simulink model "HRBModel"  (R2021b)
settings: Solver=VariableStepAuto  StartTime=0.0  StopTime=T_sim  RelTol=1e-3
values from neighbouring files (symbols this model uses):
  A = 7.20598    [HRBData.sldd]    (also in HRBModelParam.m = 7.20598)
  A_Tank = 0.25    [HRBData.sldd]    (also in HRBModelParam.m = 0.25)
  act_time = 10.0    [HRBData.sldd]    (also in HRBModelParam.m = 10)
  alpha = 0.0    [HRBData.sldd]    (also in HRBModelParam.m = deg2rad(0))
  Cd = 0.8    [HRBData.sldd]    (also in HRBModelParam.m = 0.8)
  Cr = 0.018    [HRBData.sldd]    (also in HRBModelParam.m = 0.018)
  DV = 80.0    [HRBData.sldd]    (also in HRBModelParam.m = 80)
  g = 9.81    [HRBData.sldd]    (also in HRBModelParam.m = 9.81)
  gamma = 1.4    [HRBData.sldd]    (also in HRBModelParam.m = 1.4)
  ilk_hiz = 15.0    [HRBData.sldd]    (also in HRBModelParam.m = 0)
  m = 18000.0    [HRBData.sldd]    (also in HRBModelParam.m = 18000)
  mech_eff = 0.9    [HRBData.sldd]    (also in HRBModelParam.m = 0.9)
  mu_AT = 0.8    [HRBData.sldd]    (also in HRBModelParam.m = 0.8)
  mu_HA = 0.8    [HRBData.sldd]    (also in HRBModelParam.m = 0.8)
  P0 = 50.0    [HRBData.sldd]    (also in HRBModelParam.m = 50)
  P1 = 60.0    [HRBData.sldd]    (also in HRBModelParam.m = 395)
  Patm = 1.0    [HRBData.sldd]    (also in HRBModelParam.m = 1)
  Pmax = 400.0    [HRBData.sldd]    (also in HRBModelParam.m = 400)
  r = 0.5715    [HRBData.sldd]    (also in HRBModelParam.m = 0.5715)
  R_AT = 4.11    [HRBData.sldd]    (also in HRBModelParam.m = 4.11)
  R_HA = 7.0    [HRBData.sldd]    (also in HRBModelParam.m = 7)
  R_PM_Aku = 0.07    [HRBData.sldd]    (also in HRBModelParam.m = 0.07)
  rho = 1.225    [HRBData.sldd]    (also in HRBModelParam.m = 1.225)
  rho_oil = 700.0    [HRBData.sldd]    (also in HRBModelParam.m = 700)
  V0 = 0.06    [HRBData.sldd]    (also in HRBModelParam.m = 0.06)
  V_oil = 0.1    [HRBData.sldd]    (also in HRBModelParam.m = 0.1)
  vol_eff = 0.9    [HRBData.sldd]    (also in HRBModelParam.m = 0.9)
libraries: simulink_extras x1
settings Model: DataDictionary=HRBData.sldd  Creator=erkin  LastModifiedBy=erkin

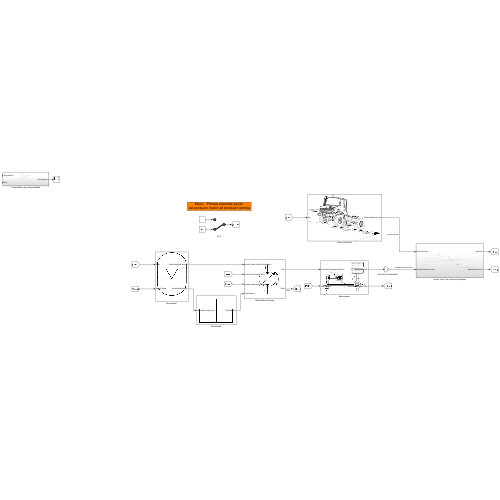
[thumbnail: Simulink's stored preview of the top-level diagram]
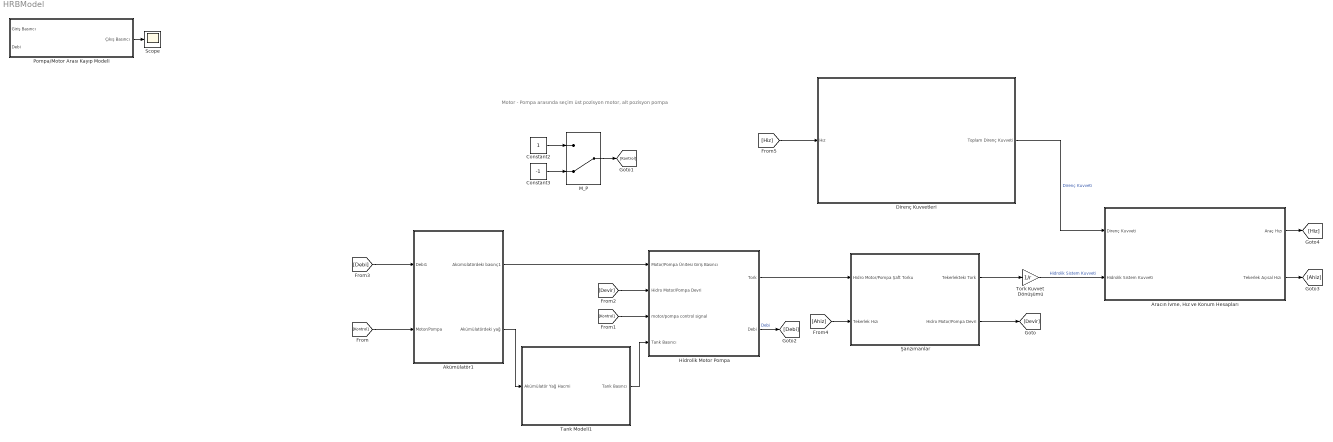
== system HRBModel ==
  note: Motor - Pompa arasında seçim
      | üst pozisyon motor, alt pozisyon pompa
  " Aracın İvme, Hız ve Konum Hesapları" : Subsystem
  Akümülatör1 : Subsystem
      mask Display: image('$imagefile'); % Use "Edit Image" on toolstrip to change.
  Constant2 : Constant
  Constant3 : Constant  Value=-1
  Direnç Kuvvetleri : Subsystem
      mask Display: image('$imagefile'); % Use "Edit Image" on toolstrip to change.
  Hidrolik Motor Pompa : Subsystem
      mask Display: image('$imagefile'); % Use "Edit Image" on toolstrip to change.
  M_P : ManualSwitch  CurrentSetting=0
  Pompa/Motor Arası Kayıp Modeli : Subsystem
  Scope : Scope
  Tank Modeli1 : Subsystem
      mask Display: image('$imagefile'); % Use "Edit Image" on toolstrip to change.
  Tork Kuvvet Dönüşümü : Gain  Gain=1/r
  Şanzımanlar : Subsystem
      mask Display: image('$imagefile'); % Use "Edit Image" on toolstrip to change.
  wires:
  Hidrolik Motor Pompa/1(Tork) -> Şanzımanlar/1(Hidro Motor/Pompa Şaft Torku)
  Şanzımanlar/1(Tekerlekteki Tork) -> Tork Kuvvet Dönüşümü/1
  Tork Kuvvet Dönüşümü/1 -> " Aracın İvme, Hız ve Konum Hesapları"/2(Hidrolik Sistem Kuvveti)  "Hidrolik Sistem Kuvveti"
  Direnç Kuvvetleri/1(Toplam Direnç Kuvveti) -> " Aracın İvme, Hız ve Konum Hesapları"/1(Direnç Kuvveti)  "Direnç Kuvveti"
  [Kontrol] -> Akümülatör1/2(Motor/Pompa)
  Constant2/1 -> M_P/1
  Constant3/1 -> M_P/2
  M_P/1 -> [Kontrol]
  [Kontrol] -> Hidrolik Motor Pompa/3(motor/pompa control signal)
  Tank Modeli1/1(Tank Basıncı) -> Hidrolik Motor Pompa/4(Tank Basıncı)
  Akümülatör1/2("Akümülatördeki yağ ") -> Tank Modeli1/1(Akümülatör Yağ Hacmi)
  Akümülatör1/1(Akümülatördeki basınç1) -> Hidrolik Motor Pompa/1(Motor/Pompa Ünitesi Giriş Basıncı)
  Pompa/Motor Arası Kayıp Modeli/1(Çıkış Basıncı) -> Scope/1
  [Devir] -> Hidrolik Motor Pompa/2(Hidro Motor/Pompa Devri)
  Şanzımanlar/2(Hidro Motor/Pompa Devri) -> [Devir]
  [Debi] -> Akümülatör1/1(Debi1)
  Hidrolik Motor Pompa/2(Debi) -> [Debi]  "Debi"
  " Aracın İvme, Hız ve Konum Hesapları"/2(Tekerlek Açısal Hızı) -> [Ahiz]
  [Ahiz] -> Şanzımanlar/2(Tekerlek Hızı)
  [Hiz] -> Direnç Kuvvetleri/1(Hız)
  " Aracın İvme, Hız ve Konum Hesapları"/1(Araç Hızı) -> [Hiz]

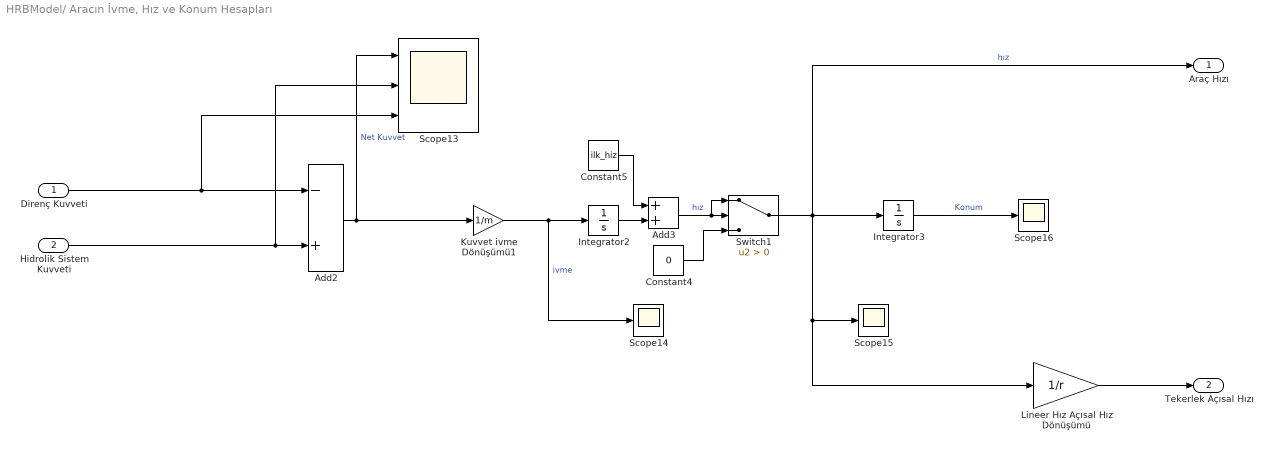
== system HRBModel/ Aracın İvme, Hız ve Konum Hesapları ==
  Direnç Kuvveti : Inport
  Hidrolik Sistem Kuvveti : Inport  Port=2
  Add2 : Sum  Inputs=-+
  Add3 : Sum
  Constant4 : Constant  Value=0
  Constant5 : Constant  Value=ilk_hiz
  Integrator2 : Integrator
  Integrator3 : Integrator
  Kuvvet ivme Dönüşümü1 : Gain  Gain=1/m
  Lineer Hız Açısal Hız Dönüşümü : Gain  Gain=1/r
  Scope13 : Scope  NumInputPorts=3
  Scope14 : Scope
  Scope15 : Scope
  Scope16 : Scope
  Switch1 : Switch  Criteria=u2 > Threshold
  Araç Hızı : Outport
  Tekerlek Açısal Hızı : Outport  Port=2
  wires:
  Kuvvet ivme Dönüşümü1/1 -> Integrator2/1, Scope14/1  "ivme"
  Constant4/1 -> Switch1/3
  Add2/1 -> Kuvvet ivme Dönüşümü1/1, Scope13/1  "Net Kuvvet"
  Integrator2/1 -> Add3/2
  Constant5/1 -> Add3/1
  Switch1/1 -> Araç Hızı/1, Integrator3/1, Lineer Hız Açısal Hız Dönüşümü/1, Scope15/1  "hız"
  Integrator3/1 -> Scope16/1  "Konum"
  Add3/1 -> Switch1/1, Switch1/2  "hız"
  Direnç Kuvveti/1 -> Scope13/3, Add2/1
  Hidrolik Sistem Kuvveti/1 -> Scope13/2, Add2/2
  Lineer Hız Açısal Hız Dönüşümü/1 -> Tekerlek Açısal Hızı/1

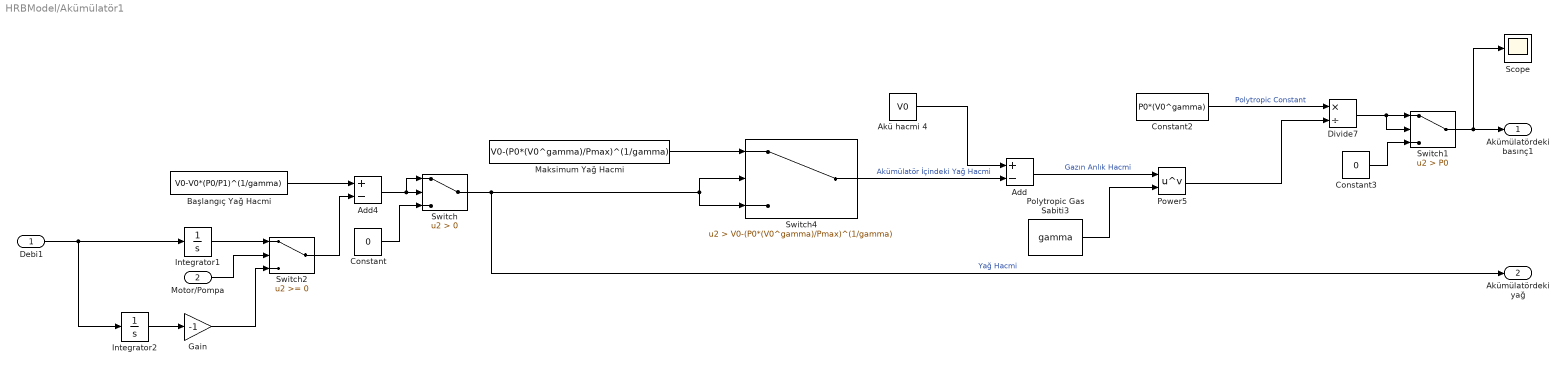
== system HRBModel/Akümülatör1 ==
  Debi1 : Inport
  Motor/Pompa : Inport  Port=2
  Add : Sum  Inputs=+-
  Add4 : Sum  Inputs=+-
  Akü hacmi 4 : Constant  Value=V0
  Başlangıç Yağ Hacmi : Constant  Value=V0-V0*(P0/P1)^(1/gamma)
  Constant : Constant  Value=0
  Constant2 : Constant  Value=P0*(V0^gamma)
  Constant3 : Constant  Value=0
  Divide7 : Product  Inputs=*/
  Gain : Gain  Gain=-1
  Integrator1 : Integrator
  Integrator2 : Integrator
  Maksimum Yağ Hacmi : Constant  Value=V0-(P0*(V0^gamma)/Pmax)^(1/gamma)
  Polytropic Gas Sabiti3 : Constant  Value=gamma
  Power5 : Math  Operator=pow  SaturateOnIntegerOverflow=on
  Scope : Scope
  Switch : Switch  Criteria=u2 > Threshold
  Switch1 : Switch  Criteria=u2 > Threshold  Threshold=P0
  Switch2 : Switch
  Switch4 : Switch  Criteria=u2 > Threshold  Threshold=V0-(P0*(V0^gamma)/Pmax)^(1/gamma)
  Akümülatördeki basınç1 : Outport
  "Akümülatördeki yağ " : Outport  Port=2
  wires:
  Divide7/1 -> Switch1/2, Switch1/1
  Başlangıç Yağ Hacmi/1 -> Add4/1
  Constant2/1 -> Divide7/1  "Polytropic Constant"
  Switch/1 -> "Akümülatördeki yağ "/1, Switch4/2, Switch4/3  "Yağ Hacmi"
  Debi1/1 -> Integrator2/1, Integrator1/1
  Akü hacmi 4/1 -> Add/1
  Add/1 -> Power5/1  "Gazın Anlık Hacmi"
  Polytropic Gas Sabiti3/1 -> Power5/2
  Power5/1 -> Divide7/2
  Add4/1 -> Switch/1, Switch/2
  Constant/1 -> Switch/3
  Constant3/1 -> Switch1/3
  Integrator1/1 -> Switch2/1
  Switch2/1 -> Add4/2
  Integrator2/1 -> Gain/1
  Gain/1 -> Switch2/3
  Switch1/1 -> Scope/1, Akümülatördeki basınç1/1
  Motor/Pompa/1 -> Switch2/2
  Maksimum Yağ Hacmi/1 -> Switch4/1
  Switch4/1 -> Add/2  "Akümülatör İçindeki Yağ Hacmi"

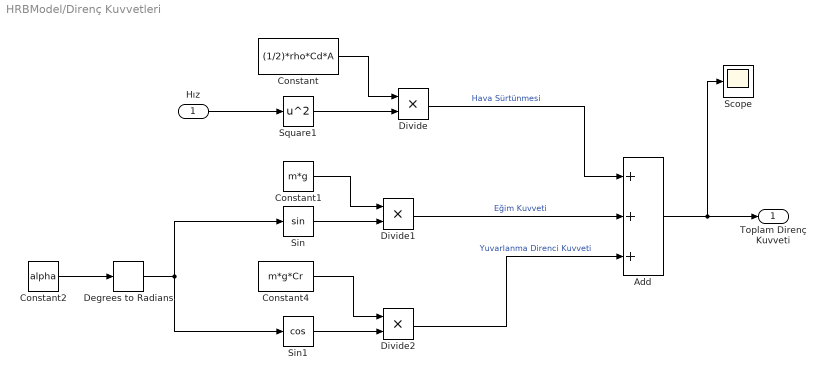
== system HRBModel/Direnç Kuvvetleri ==
  Hız : Inport
  Add : Sum  Inputs=+++
  Constant : Constant  Value=(1/2)*rho*Cd*A
  Constant1 : Constant  Value=m*g
  Constant2 : Constant  Value=alpha
  Constant4 : Constant  Value=m*g*Cr
  Degrees to Radians : simulink_extras/Transformations/Degrees to Radians
  Divide : Product  Inputs=**
  Divide1 : Product  Inputs=**
  Divide2 : Product  Inputs=**
  Scope : Scope
  Sin : Trigonometry
  Sin1 : Trigonometry  Operator=cos
  Square1 : Math  Operator=square  SaturateOnIntegerOverflow=on
  Toplam Direnç Kuvveti : Outport
  wires:
  Sin1/1 -> Divide2/2
  Divide1/1 -> Add/2  "Eğim Kuvveti"
  Divide2/1 -> Add/3  "Yuvarlanma Direnci Kuvveti"
  Add/1 -> Scope/1, Toplam Direnç Kuvveti/1
  Hız/1 -> Square1/1
  Constant2/1 -> Degrees to Radians/1
  Degrees to Radians/1 -> Sin1/1, Sin/1
  Square1/1 -> Divide/2
  Constant/1 -> Divide/1
  Divide/1 -> Add/1  "Hava Sürtünmesi"
  Constant1/1 -> Divide1/1
  Sin/1 -> Divide1/2
  Constant4/1 -> Divide2/1

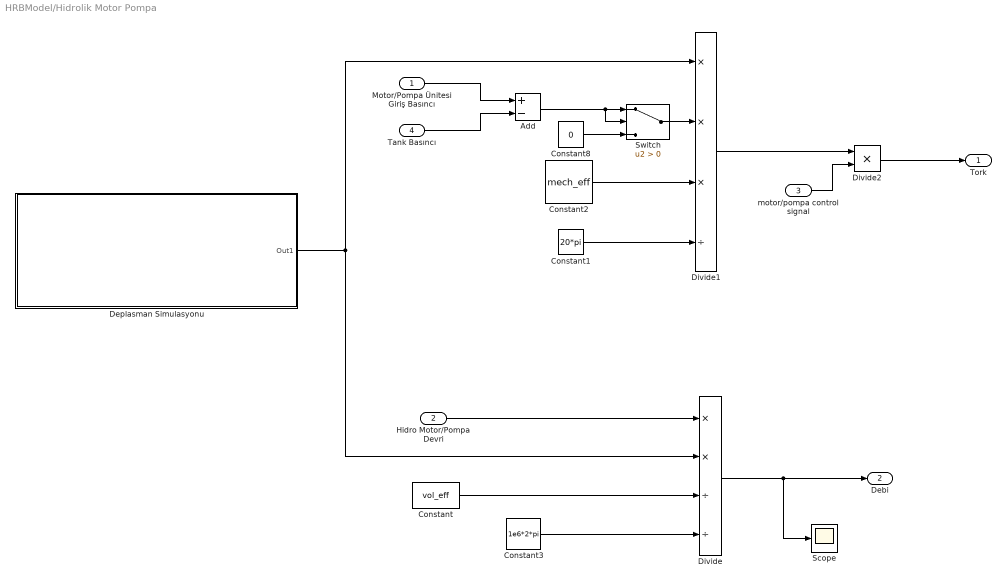
== system HRBModel/Hidrolik Motor Pompa ==
  Motor/Pompa Ünitesi Giriş Basıncı : Inport
  Hidro Motor/Pompa Devri : Inport  Port=2
  motor/pompa control signal : Inport  Port=3
  Tank Basıncı : Inport  Port=4
  Add : Sum  Inputs=+-
  Constant : Constant  Value=vol_eff
  Constant1 : Constant  Value=20*pi
  Constant2 : Constant  Value=mech_eff
  Constant3 : Constant  Value=1e6*2*pi
  Constant8 : Constant  Value=0
  Deplasman Simulasyonu : Subsystem
  Divide : Product  Inputs=**//
  Divide1 : Product  Inputs=***/
  Divide2 : Product  Inputs=**
  Scope : Scope
  Switch : Switch  Criteria=u2 > Threshold
  Tork : Outport
  Debi : Outport  Port=2
  wires:
  Constant1/1 -> Divide1/4
  Constant2/1 -> Divide1/3
  Motor/Pompa Ünitesi Giriş Basıncı/1 -> Add/1
  Divide1/1 -> Divide2/1
  Hidro Motor/Pompa Devri/1 -> Divide/1
  Constant/1 -> Divide/3
  Divide/1 -> Scope/1, Debi/1
  Constant3/1 -> Divide/4
  Divide2/1 -> Tork/1
  motor/pompa control signal/1 -> Divide2/2
  Add/1 -> Switch/2, Switch/1
  Switch/1 -> Divide1/2
  Constant8/1 -> Switch/3
  Tank Basıncı/1 -> Add/2
  Deplasman Simulasyonu/1(Out1) -> Divide1/1, Divide/2

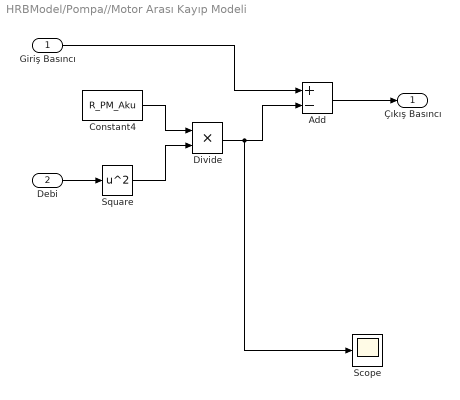
== system HRBModel/Pompa//Motor Arası Kayıp Modeli ==
  Giriş Basıncı : Inport
  Debi : Inport  Port=2
  Add : Sum  Inputs=+-
  Constant4 : Constant  Value=R_PM_Aku
  Divide : Product  Inputs=**
  Scope : Scope
  Square : Math  Operator=square  SaturateOnIntegerOverflow=on
  Çıkış Basıncı : Outport
  wires:
  Debi/1 -> Square/1
  Square/1 -> Divide/2
  Constant4/1 -> Divide/1
  Giriş Basıncı/1 -> Add/1
  Divide/1 -> Scope/1, Add/2
  Add/1 -> Çıkış Basıncı/1

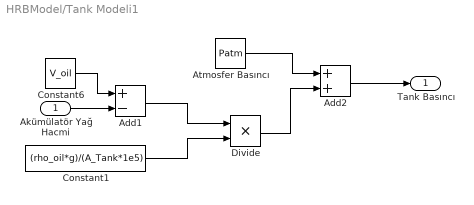
== system HRBModel/Tank Modeli1 ==
  Akümülatör Yağ Hacmi : Inport
  Add1 : Sum  Inputs=+-
  Add2 : Sum
  Atmosfer Basıncı : Constant  Value=Patm
  Constant1 : Constant  Value=(rho_oil*g)/(A_Tank*1e5)
  Constant6 : Constant  Value=V_oil
  Divide : Product  Inputs=**
  Tank Basıncı : Outport
  wires:
  Constant6/1 -> Add1/1
  Add1/1 -> Divide/1
  Akümülatör Yağ Hacmi/1 -> Add1/2
  Atmosfer Basıncı/1 -> Add2/1
  Add2/1 -> Tank Basıncı/1
  Constant1/1 -> Divide/2
  Divide/1 -> Add2/2

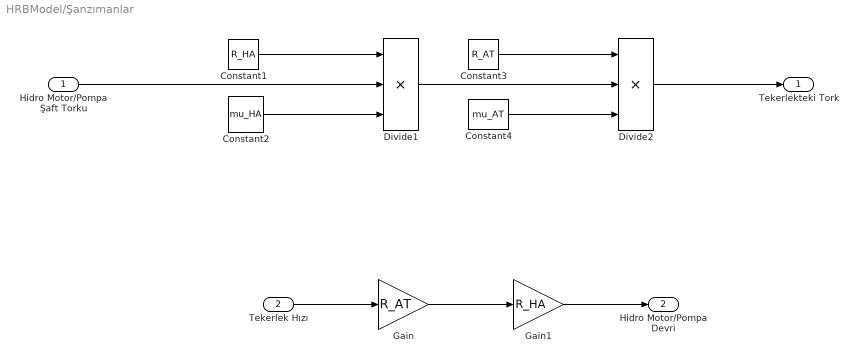
== system HRBModel/Şanzımanlar ==
  Hidro Motor/Pompa Şaft Torku : Inport
  Tekerlek Hızı : Inport  Port=2
  Constant1 : Constant  Value=R_HA
  Constant2 : Constant  Value=mu_HA
  Constant3 : Constant  Value=R_AT
  Constant4 : Constant  Value=mu_AT
  Divide1 : Product  Inputs=***
  Divide2 : Product  Inputs=***
  Gain : Gain  Gain=R_AT
  Gain1 : Gain  Gain=R_HA
  Tekerlekteki Tork : Outport
  Hidro Motor/Pompa Devri : Outport  Port=2
  wires:
  Constant3/1 -> Divide2/1
  Constant2/1 -> Divide1/3
  Divide2/1 -> Tekerlekteki Tork/1
  Constant4/1 -> Divide2/3
  Constant1/1 -> Divide1/1
  Divide1/1 -> Divide2/2
  Hidro Motor/Pompa Şaft Torku/1 -> Divide1/2
  Tekerlek Hızı/1 -> Gain/1
  Gain/1 -> Gain1/1
  Gain1/1 -> Hidro Motor/Pompa Devri/1

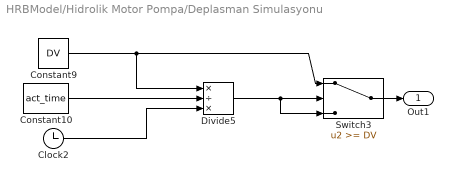
== system HRBModel/Hidrolik Motor Pompa/Deplasman Simulasyonu ==
  Clock2 : Clock
  Constant10 : Constant  Value=act_time
  Constant9 : Constant  Value=DV
  Divide5 : Product  Inputs=*/*
  Switch3 : Switch  Threshold=DV
  Out1 : Outport
  wires:
  Clock2/1 -> Divide5/3
  Divide5/1 -> Switch3/3, Switch3/2
  Switch3/1 -> Out1/1
  Constant9/1 -> Divide5/1, Switch3/1
  Constant10/1 -> Divide5/2
